simulink model "BoundedTorqueControlR2016bS88"  (Simulink 8.8)
settings: Solver=FixedStepDiscrete  StartTime=0.0  StopTime=CONFIG.SIMULATION_TIME  FixedStep=CONFIG.Ts  RelTol=1e-3  EnableMultiTasking=on
InitFcn:
  | cd(fileparts(which(bdroot)));
  | init_BoundedTorqueControl;
undefined symbols (not defined in the file or in its folder): CONFIG, DiscIntNeverNeededParam, model, ROBOT_DOF, sat
libraries: WBToolboxLibrary x12
settings Model: SuppressorTable=22 serialization::archive 11 0 6 0 0 0 11 0  Creator=marie  LastModifiedBy=mcharbonneau
settings DataIOCC: SaveFormat=Dataset  SignalLoggingSaveFormat=Dataset
settings DebuggingCC: UnderspecifiedInitializationDetection=Simplified  MergeDetectMultiDrivingBlocksExec=error  FcnCallInpInsideContextMsg=error  AllowSymbolicDim=off  StateNameClashWarn=none
settings HardwareCC: ProdBitPerPointer=64  ProdBitPerSizeT=64  ProdBitPerPtrDiffT=64  ProdLargestAtomicFloat=Float  ProdIntDivRoundTo=Zero  ProdEndianess=LittleEndian  ProdWordSize=64  ProdHWDeviceType=Intel->x86-64 (Windows64)
settings GRTTargetCC: GeneratePreprocessorConditionals=Use local settings  CombineOutputUpdateFcns=on  GRTInterface=off

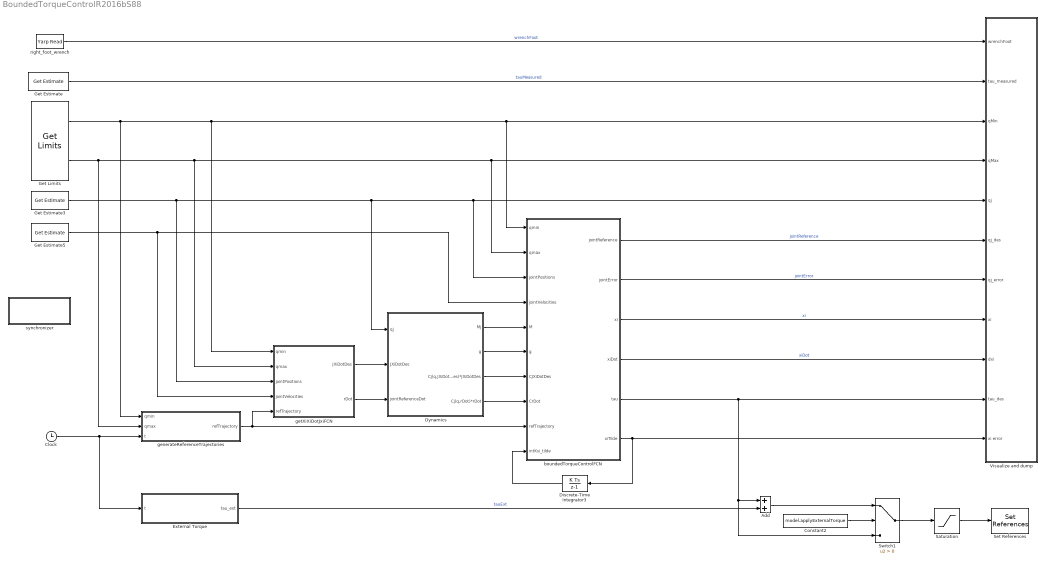
== system BoundedTorqueControlR2016bS88 ==
  Add : Sum
  Clock : Clock
  Constant2 : Constant  Value=model.applyExternalTorque
  Discrete-Time Integrator3 : DiscreteIntegrator  InitialCondition=zeros(ROBOT_DOF,1)  InitialConditionSetting=State (most efficient)  SampleTime=CONFIG.Ts  ICPrevOutput=DiscIntNeverNeededParam  ICPrevScaledInput=DiscIntNeverNeededParam
  Dynamics : Subsystem
  External Torque : MATLAB Function  TreatAsAtomicUnit=on
  Get Estimate : WBToolboxLibrary/wholeBodyStates/Get Estimate  estimateType=Joints Torque  robotName=WBT_robotName  localName=WBT_modelName  wbiFile=WBT_wbiFilename  wbiList=WBT_wbiList
  Get Estimate3 : WBToolboxLibrary/wholeBodyStates/Get Estimate  estimateType=Joints Position  robotName=WBT_robotName  localName=WBT_modelName  wbiFile=WBT_wbiFilename  wbiList=WBT_wbiList
  Get Estimate5 : WBToolboxLibrary/wholeBodyStates/Get Estimate  estimateType=Joints Velocity  robotName=WBT_robotName  localName=WBT_modelName  wbiFile=WBT_wbiFilename  wbiList=WBT_wbiList
  Get Limits : WBToolboxLibrary/wholeBodyStates/Get Limits  limitsType=Position  robotName=WBT_robotName  localName=WBT_modelName  wbiFile=WBT_wbiFilename  wbiList=WBT_wbiList
  Saturation : Saturate  UpperLimit=sat.torque  LowerLimit=-sat.torque
  Set References : WBToolboxLibrary/wholeBodyActuators/Set References  controlType=Torque  fullOrSubControl=Full  controlledJoints=''  robotName=WBT_robotName  localName=WBT_modelName  wbiFile=WBT_wbiFilename  wbiList=WBT_wbiList
  Switch1 : Switch  Criteria=u2 > Threshold
  Visualize and dump : Subsystem
  boundedTorqueControlFCN : MATLAB Function  TreatAsAtomicUnit=on
  generateReferenceTrajectories : MATLAB Function  TreatAsAtomicUnit=on
  getXiXiDotJxiFCN : MATLAB Function  TreatAsAtomicUnit=on
  right_foot_wrench : WBToolboxLibrary/Utilities/Yarp Read  portName=PORTS.WBDT_RIGHTLEG_EE  signalSize=6  blocking=off  timestamp=off  autoconnect=on  errorOnConnection=on
  synchronizer : Subsystem
      mask Display: disp('SYNCHRONIZER')
  wires:
  Get Estimate3/1 -> boundedTorqueControlFCN/3(jointPositions), Visualize and dump/5(qj), Dynamics/1(qj), getXiXiDotJxiFCN/3(jointPositions)
  Get Estimate5/1 -> boundedTorqueControlFCN/4(jointVelocities), getXiXiDotJxiFCN/4(jointVelocities)
  Dynamics/1(Mj) -> boundedTorqueControlFCN/5(M)
  Get Limits/2 -> boundedTorqueControlFCN/2(qmax), Visualize and dump/4(qMax), getXiXiDotJxiFCN/2(qmax), generateReferenceTrajectories/2(qmax)
  Get Limits/1 -> generateReferenceTrajectories/1(qmin), boundedTorqueControlFCN/1(qmin), Visualize and dump/3(qMin), getXiXiDotJxiFCN/1(qmin)
  boundedTorqueControlFCN/5(tau) -> Switch1/3, Add/1, Visualize and dump/10(tau_des)
  Discrete-Time Integrator3/1 -> boundedTorqueControlFCN/10(intKsi_tilde)
  Clock/1 -> generateReferenceTrajectories/3(t), External Torque/1(t)
  External Torque/1(tau_ext) -> Add/2  "tauExt"
  generateReferenceTrajectories/1(refTrajectory) -> boundedTorqueControlFCN/9(refTrajectory), getXiXiDotJxiFCN/5(refTrajectory)
  Dynamics/2(g) -> boundedTorqueControlFCN/6(g)
  getXiXiDotJxiFCN/1(JXiDotDes) -> Dynamics/2(JXiDotDes)
  Dynamics/3(Cj(q,JXiDotDes)*JXiDotDes) -> boundedTorqueControlFCN/7(CJXiDotDes)
  boundedTorqueControlFCN/6(xiTilde) -> Visualize and dump/11(xi error), Discrete-Time Integrator3/1
  getXiXiDotJxiFCN/2(rDot) -> Dynamics/3(jointReferenceDot)
  Dynamics/4(Cj(q,rDot)*rDot) -> boundedTorqueControlFCN/8(CrDot)
  Add/1 -> Switch1/1
  Switch1/1 -> Saturation/1
  Constant2/1 -> Switch1/2
  Get Estimate/1 -> Visualize and dump/2(tau_measured)  "tauMeasured"
  right_foot_wrench/1 -> Visualize and dump/1(wrenchFoot)  "wrenchFoot"
  boundedTorqueControlFCN/4(xiDot) -> Visualize and dump/9(dxi)  "xiDot"
  boundedTorqueControlFCN/1(jointReference) -> Visualize and dump/6(qj_des)  "jointReference"
  boundedTorqueControlFCN/2(jointError) -> Visualize and dump/7(qj_error)  "jointError"
  boundedTorqueControlFCN/3(xi) -> Visualize and dump/8(xi)  "xi"
  Saturation/1 -> Set References/1

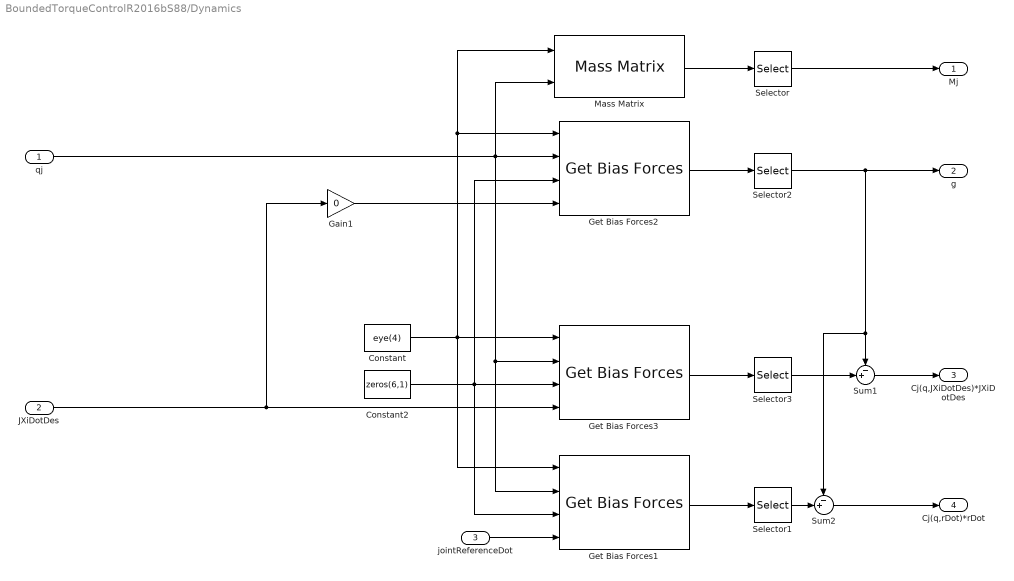
== system BoundedTorqueControlR2016bS88/Dynamics ==
  qj : Inport
  JXiDotDes : Inport  Port=2
  jointReferenceDot : Inport  Port=3
  Constant : Constant  Value=eye(4)
  Constant2 : Constant  Value=zeros(6,1)
  Gain1 : Gain  Gain=0
  Get Bias Forces1 : WBToolboxLibrary/wholeBodyModel/Dynamics/Get Bias Forces  robotName=WBT_robotName  localName=WBT_modelName  wbiFile=WBT_wbiFilename  wbiList=WBT_wbiList  explicitGravity=off
  Get Bias Forces2 : WBToolboxLibrary/wholeBodyModel/Dynamics/Get Bias Forces  robotName=WBT_robotName  localName=WBT_modelName  wbiFile=WBT_wbiFilename  wbiList=WBT_wbiList  explicitGravity=off
  Get Bias Forces3 : WBToolboxLibrary/wholeBodyModel/Dynamics/Get Bias Forces  robotName=WBT_robotName  localName=WBT_modelName  wbiFile=WBT_wbiFilename  wbiList=WBT_wbiList  explicitGravity=off
  Mass Matrix : WBToolboxLibrary/wholeBodyModel/Dynamics/Mass Matrix  robotName=WBT_robotName  localName=WBT_modelName  wbiFile=WBT_wbiFilename  wbiList=WBT_wbiList
  Selector : Selector  NumberOfDimensions=2  InputPortWidth=3  IndexOptions=Index vector (dialog),Index vector (dialog)  Indices=[7:6+ROBOT_DOF],[7:6+ROBOT_DOF]  OutputSizes=1,1
  Selector1 : Selector  InputPortWidth=ROBOT_DOF+6  IndexOptions=Index vector (dialog)  Indices=[7:ROBOT_DOF+6]  OutputSizes=1
  Selector2 : Selector  InputPortWidth=ROBOT_DOF+6  IndexOptions=Index vector (dialog)  Indices=[7:ROBOT_DOF+6]  OutputSizes=1
  Selector3 : Selector  InputPortWidth=ROBOT_DOF+6  IndexOptions=Index vector (dialog)  Indices=[7:ROBOT_DOF+6]  OutputSizes=1
  Sum1 : Sum  Inputs=-+|
  Sum2 : Sum  Inputs=-+|
  Mj : Outport
  g : Outport  Port=2
  Cj(q,JXiDotDes)*JXiDotDes : Outport  Port=3
  Cj(q,rDot)*rDot : Outport  Port=4
  wires:
  Constant2/1 -> Get Bias Forces2/3, Get Bias Forces1/3, Get Bias Forces3/3
  Get Bias Forces2/1 -> Selector2/1
  Get Bias Forces3/1 -> Selector3/1
  Selector3/1 -> Sum1/2
  Sum1/1 -> Cj(q,JXiDotDes)*JXiDotDes/1
  JXiDotDes/1 -> Gain1/1, Get Bias Forces3/4
  Selector/1 -> Mj/1
  qj/1 -> Mass Matrix/2, Get Bias Forces1/2, Get Bias Forces3/2, Get Bias Forces2/2
  Mass Matrix/1 -> Selector/1
  Constant/1 -> Get Bias Forces2/1, Mass Matrix/1, Get Bias Forces1/1, Get Bias Forces3/1
  jointReferenceDot/1 -> Get Bias Forces1/4
  Selector2/1 -> Sum2/1, Sum1/1, g/1
  Selector1/1 -> Sum2/2
  Sum2/1 -> Cj(q,rDot)*rDot/1
  Get Bias Forces1/1 -> Selector1/1
  Gain1/1 -> Get Bias Forces2/4

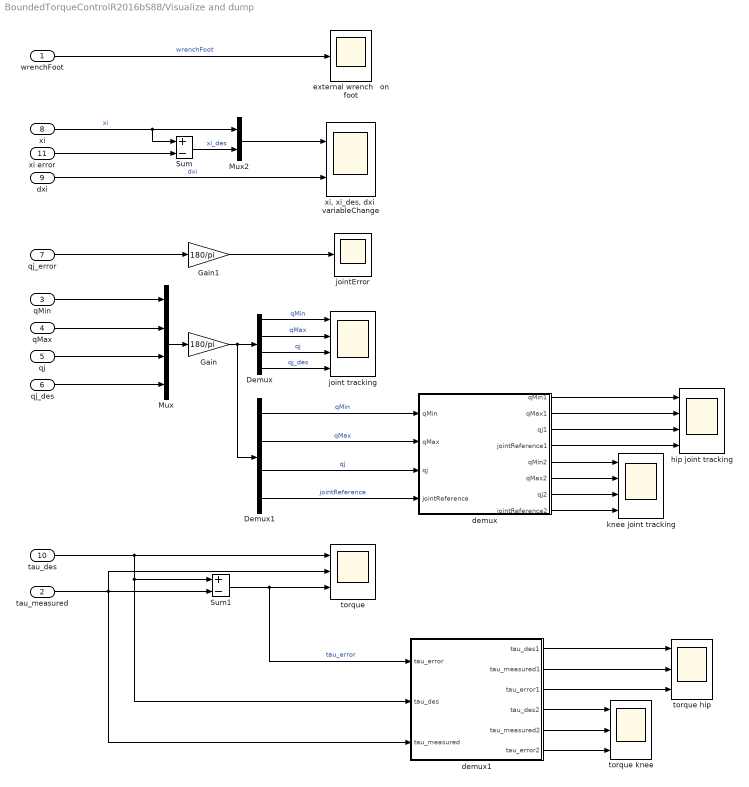
== system BoundedTorqueControlR2016bS88/Visualize and dump ==
  wrenchFoot : Inport
  tau_measured : Inport  Port=2
  qMin : Inport  Port=3
  qMax : Inport  Port=4
  qj : Inport  Port=5
  qj_des : Inport  Port=6
  qj_error : Inport  Port=7
  xi : Inport  Port=8
  dxi : Inport  Port=9
  tau_des : Inport  Port=10
  xi error : Inport  Port=11
  Demux : Demux
  Demux1 : Demux
  Gain : Gain  Gain=180/pi
  Gain1 : Gain  Gain=180/pi
  Mux : Mux
  Mux2 : Mux  Inputs=2
  Sum : Sum  Inputs=+-
  Sum1 : Sum  Inputs=+-
  demux : MATLAB Function  TreatAsAtomicUnit=on
  demux1 : MATLAB Function  TreatAsAtomicUnit=on
  external wrench   on foot : Scope
  hip joint tracking : Scope  NumInputPorts=4
  joint tracking : Scope  NumInputPorts=4
  jointError : Scope
  knee joint tracking : Scope  NumInputPorts=4
  torque : Scope  NumInputPorts=3
  torque hip : Scope  NumInputPorts=3
  torque knee : Scope  NumInputPorts=3
  "xi, xi_des, dxi  variableChange" : Scope  NumInputPorts=2
  wires:
  xi error/1 -> Sum/2
  dxi/1 -> "xi, xi_des, dxi  variableChange"/2  "dxi"
  Sum/1 -> Mux2/2  "xi_des"
  xi/1 -> Sum/1, Mux2/1  "xi"
  Mux2/1 -> "xi, xi_des, dxi  variableChange"/1
  Demux/4 -> joint tracking/4  "qj_des"
  Demux/2 -> joint tracking/2  "qMax"
  Demux/3 -> joint tracking/3  "qj"
  Demux/1 -> joint tracking/1  "qMin"
  qMin/1 -> Mux/1
  qMax/1 -> Mux/2
  qj/1 -> Mux/3
  qj_des/1 -> Mux/4
  Mux/1 -> Gain/1
  Gain/1 -> Demux1/1, Demux/1
  Gain1/1 -> jointError/1
  qj_error/1 -> Gain1/1
  Demux1/1 -> demux/1(qMin)  "qMin"
  demux/8(jointReference2) -> knee joint tracking/4
  demux/6(qMax2) -> knee joint tracking/2
  Demux1/2 -> demux/2(qMax)  "qMax"
  demux/5(qMin2) -> knee joint tracking/1
  demux/4(jointReference1) -> hip joint tracking/4
  Demux1/3 -> demux/3(qj)  "qj"
  Demux1/4 -> demux/4(jointReference)  "jointReference"
  demux/3(qj1) -> hip joint tracking/3
  demux/7(qj2) -> knee joint tracking/3
  demux/1(qMin1) -> hip joint tracking/1
  demux/2(qMax1) -> hip joint tracking/2
  Sum1/1 -> demux1/1(tau_error), torque/3  "tau_error"
  tau_des/1 -> torque/1, demux1/2(tau_des), Sum1/1
  tau_measured/1 -> Sum1/2, demux1/3(tau_measured), torque/2
  wrenchFoot/1 -> external wrench   on foot/1  "wrenchFoot"
  demux1/2(tau_measured1) -> torque hip/2
  demux1/5(tau_measured2) -> torque knee/2
  demux1/1(tau_des1) -> torque hip/1
  demux1/6(tau_error2) -> torque knee/3
  demux1/4(tau_des2) -> torque knee/1
  demux1/3(tau_error1) -> torque hip/3

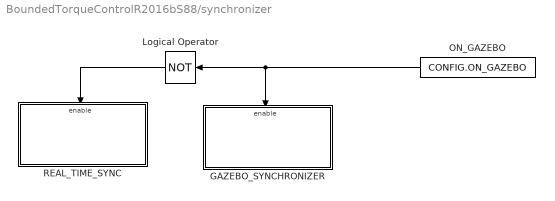
== system BoundedTorqueControlR2016bS88/synchronizer ==
  GAZEBO_SYNCHRONIZER : Subsystem
  Logical Operator : Logic  Operator=NOT  AllPortsSameDT=off  OutDataTypeStr=boolean
  "ON_GAZEBO " : Constant  Value=CONFIG.ON_GAZEBO
  REAL_TIME_SYNC : Subsystem
  wires:
  Logical Operator/1 -> REAL_TIME_SYNC/Enable
  "ON_GAZEBO "/1 -> GAZEBO_SYNCHRONIZER/Enable, Logical Operator/1

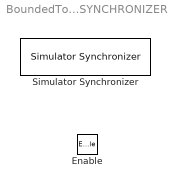
== system BoundedTorqueControlR2016bS88/synchronizer/GAZEBO_SYNCHRONIZER ==
  Enable : EnablePort
  Simulator Synchronizer : WBToolboxLibrary/Utilities/Simulator Synchronizer  period=CONFIG.Ts  serverPortName='/clock/rpc'  clientPortName='/WBT_synchronizer/rpc:o'

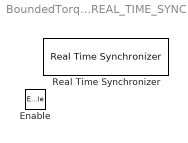
== system BoundedTorqueControlR2016bS88/synchronizer/REAL_TIME_SYNC ==
  Enable : EnablePort
  Real Time Synchronizer : WBToolboxLibrary/Utilities/Real Time Synchronizer  period=CONFIG.Ts

== matlab function boundedTorqueControlFCN ==
  data: jointReference output double; jointError output double; xi output double; xiDot output double; tau output double; xiTilde output double; model parameter double; qmin input double; qmax input double; jointPositions input double; jointVelocities input double; M input double; g input double; CJXiDotDes input double; CrDot input double; refTrajectory input double; intKsi_tilde input double
function [jointReference, jointError, xi, xiDot, tau, xiTilde] =  boundedJointEvolutionControl(model, qmin, qmax, jointPositions, jointVelocities, M, g, CJXiDotDes, CrDot, refTrajectory, intKsi_tilde)


    [jointReference, jointError, xi, xiDot, tau, xiTilde] = boundedJointEvolutionControl(model, qmin, qmax, jointPositions, jointVelocities, M, g, CJXiDotDes, CrDot,  refTrajectory, intKsi_tilde);

== matlab function generateReferenceTrajectories ==
  data: qmin input double; qmax input double; refTrajectory output double; t input double; model parameter double; ROBOT_DOF parameter double
 function refTrajectory  = generateReferenceTrajectoriesFCN(qmin,qmax, t, model,ROBOT_DOF)

refTrajectory  = generateReferenceTrajectories(qmin,qmax, t, model, ROBOT_DOF);

== matlab function External Torque ==
  data: tau_ext output double; t input double; model parameter double
function tau_ext = applyExternTorqueFCN(t, model)

tau_ext = applyExternTorque(t, model);

== matlab function getXiXiDotJxiFCN ==
  data: qmin input double; qmax input double; JXiDotDes output double; jointPositions input double; jointVelocities input double; refTrajectory input double; rDot output double
function [JXiDotDes,rDot]  = variableChange(qmin, qmax, jointPositions, jointVelocities, refTrajectory)


[~,~,J,~]        = getXiXiDotJxi(jointPositions, jointVelocities, qmin, qmax);

[r,rDot,~]       = getReferences(refTrajectory);

[~,xiDotDes,~,~] = getXiXiDotJxi(r,rDot,qmin, qmax);

JXiDotDes        = J*xiDotDes;

== matlab function Visualize and dump/demux1 ==
  data: tau_error input double; tau_des input double; tau_measured input double; tau_des1 output double; tau_measured1 output double; tau_error1 output double; tau_des2 output double; tau_measured2 output double; tau_error2 output double
function [tau_des1, tau_measured1, tau_error1, tau_des2, tau_measured2, tau_error2]  = demux_tau(tau_error, tau_des, tau_measured)

tau_des1 = tau_des(1);
tau_measured1 = tau_measured(1);
tau_error1 = tau_error(1);

tau_des2 = tau_des(2);
tau_measured2 = tau_measured(2);
tau_error2 = tau_error(2);

== matlab function Visualize and dump/demux ==
  data: qMin1 output double; qMin input double; qMax input double; qj input double; jointReference input double; qMax1 output double; qj1 output double; jointReference1 output double; qMin2 output double; qMax2 output double; qj2 output double; jointReference2 output double
function [qMin1, qMax1, qj1, jointReference1, qMin2, qMax2, qj2, jointReference2]  = demux_q(qMin,qMax, qj, jointReference)

qMin1 = qMin(1);
qMax1 = qMax(1);
qj1 = qj(1);
jointReference1 = jointReference(1);

qMin2 = qMin(2);
qMax2 = qMax(2);
qj2 = qj(2);
jointReference2 = jointReference(2);
